simulink subsystem "sensorDynamics"  (R2021a)
settings: Solver=VariableStepAuto  StartTime=0.0  StopTime=10.0  RelTol=1e-3
settings Model: Creator=Laura  LastModifiedBy=Laura

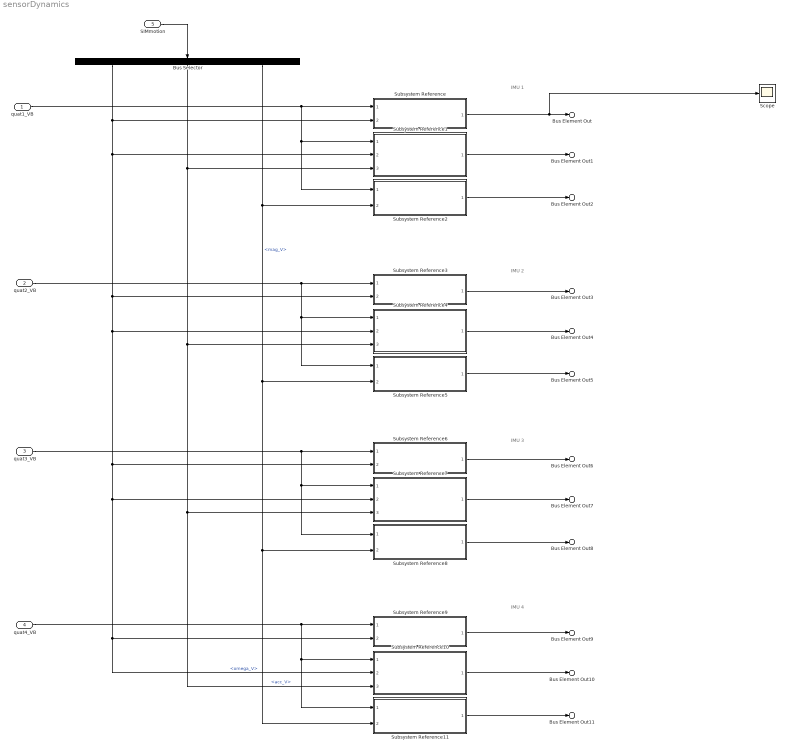
== system sensorDynamics ==
  note: IMU 1
  note: IMU 4
  note: IMU 3
  note: IMU 2
  quat1_VB : Inport
  quat2_VB : Inport  Port=2
  quat3_VB : Inport  Port=3
  quat4_VB : Inport  Port=4
  SIMmotion : Inport  Port=5
  Bus Selector : BusSelector  OutputSignals=omega_V,acc_V,mag_V
  Scope : Scope
  Subsystem Reference{,3,6,9} (4 alike) : Subsystem  ReferencedSubsystem=gyroCM2Sensor
  Subsystem Reference{1,4,7,10} (4 alike) : Subsystem  ReferencedSubsystem=accCM2Sensor
  Subsystem Reference{2,5,8,11} (4 alike) : Subsystem  ReferencedSubsystem=magCM2Sensor
  Bus Element Out : Outport  PortName=SensorDynamics  Element=omega_B1
  Bus Element Out3 : Outport  PortName=SensorDynamics  Element=omega_B2
  Bus Element Out6 : Outport  PortName=SensorDynamics  Element=omega_B3
  Bus Element Out9 : Outport  PortName=SensorDynamics  Element=omega_B4
  Bus Element Out1 : Outport  PortName=SensorDynamics  Element=acc_B1
  Bus Element Out4 : Outport  PortName=SensorDynamics  Element=acc_B2
  Bus Element Out7 : Outport  PortName=SensorDynamics  Element=acc_B3
  Bus Element Out10 : Outport  PortName=SensorDynamics  Element=acc_B4
  Bus Element Out2 : Outport  PortName=SensorDynamics  Element=mag_B1
  Bus Element Out5 : Outport  PortName=SensorDynamics  Element=mag_B2
  Bus Element Out8 : Outport  PortName=SensorDynamics  Element=mag_B3
  Bus Element Out11 : Outport  PortName=SensorDynamics  Element=mag_B4
  wires:
  Subsystem Reference10/1 -> Bus Element Out10/1
  Subsystem Reference/1 -> Bus Element Out/1, Scope/1
  Subsystem Reference11/1 -> Bus Element Out11/1
  Subsystem Reference4/1 -> Bus Element Out4/1
  Subsystem Reference7/1 -> Bus Element Out7/1
  quat3_VB/1 -> Subsystem Reference8/1, Subsystem Reference7/1, Subsystem Reference6/1
  Bus Selector/3 -> Subsystem Reference5/2, Subsystem Reference11/2, Subsystem Reference8/2, Subsystem Reference2/2  "<mag_V>"
  Subsystem Reference5/1 -> Bus Element Out5/1
  quat2_VB/1 -> Subsystem Reference5/1, Subsystem Reference4/1, Subsystem Reference3/1
  Subsystem Reference6/1 -> Bus Element Out6/1
  quat1_VB/1 -> Subsystem Reference2/1, Subsystem Reference1/1, Subsystem Reference/1
  Bus Selector/2 -> Subsystem Reference1/3, Subsystem Reference4/3, Subsystem Reference10/3, Subsystem Reference7/3  "<acc_V>"
  SIMmotion/1 -> Bus Selector/1
  Bus Selector/1 -> Subsystem Reference/2, Subsystem Reference9/2, Subsystem Reference10/2, Subsystem Reference7/2, Subsystem Reference6/2, Subsystem Reference4/2, Subsystem Reference3/2, Subsystem Reference1/2  "<omega_V>"
  Subsystem Reference3/1 -> Bus Element Out3/1
  Subsystem Reference9/1 -> Bus Element Out9/1
  Subsystem Reference1/1 -> Bus Element Out1/1
  quat4_VB/1 -> Subsystem Reference11/1, Subsystem Reference10/1, Subsystem Reference9/1
  Subsystem Reference8/1 -> Bus Element Out8/1
  Subsystem Reference2/1 -> Bus Element Out2/1
